simulink model "dynamicIMmodel"  (R2023b)
settings: Solver=VariableStepAuto  StartTime=0.0  StopTime=100  RelTol=1e-3
undefined symbols (not defined in the file): J, P, rr, rs, wb, Wb, We, Xlr, Xls, Xm
settings Model: Creator=Akaashdeep B  LastModifiedBy=Akaashdeep B

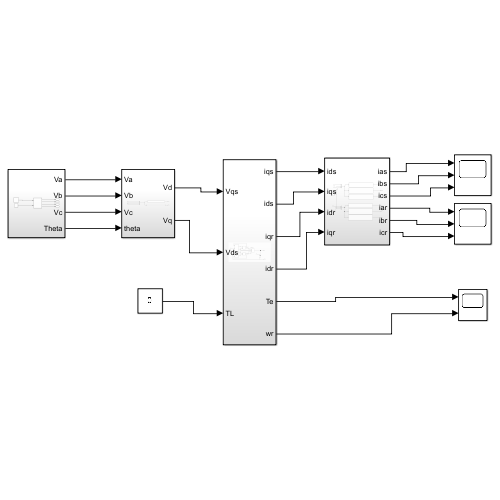
[thumbnail: Simulink's stored preview of the top-level diagram]
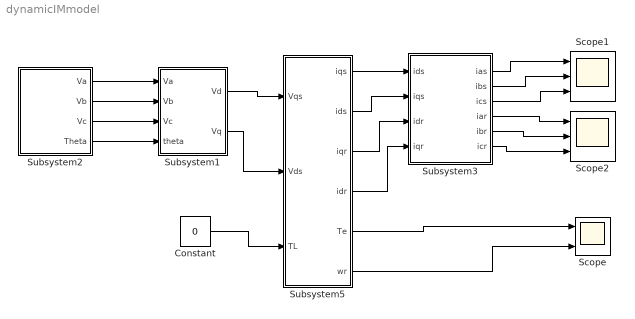
== system dynamicIMmodel ==
  Constant : Constant  Value=0
  Scope : Scope  NumInputPorts=2
  Scope1 : Scope  NumInputPorts=3
  Scope2 : Scope  NumInputPorts=3
  Subsystem1 : Subsystem
  Subsystem2 : Subsystem
  Subsystem3 : Subsystem
  Subsystem5 : Subsystem
  wires:
  Subsystem2/1(Va) -> Subsystem1/1(Va)
  Subsystem2/2(Vb) -> Subsystem1/2(Vb)
  Subsystem2/4(Theta) -> Subsystem1/4(theta)
  Subsystem1/1(Vd) -> Subsystem5/1(Vqs)
  Subsystem1/2(Vq) -> Subsystem5/2(Vds)
  Constant/1 -> Subsystem5/3(TL)
  Subsystem5/6(wr) -> Scope/2
  Subsystem5/5(Te) -> Scope/1
  Subsystem5/1(iqs) -> Subsystem3/1(ids)
  Subsystem5/2(ids) -> Subsystem3/2(iqs)
  Subsystem5/3(iqr) -> Subsystem3/3(idr)
  Subsystem5/4(idr) -> Subsystem3/4(iqr)
  Subsystem3/1(ias) -> Scope1/1
  Subsystem3/2(ibs) -> Scope1/2
  Subsystem3/3(ics) -> Scope1/3
  Subsystem3/4(iar) -> Scope2/1
  Subsystem3/5(ibr) -> Scope2/2
  Subsystem3/6(icr) -> Scope2/3
  Subsystem2/3(Vc) -> Subsystem1/3(Vc)

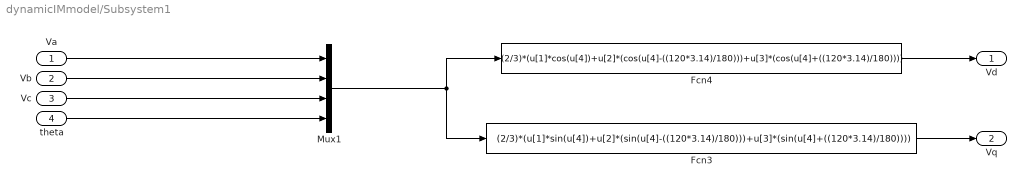
== system dynamicIMmodel/Subsystem1 ==
  Va : Inport
  Vb : Inport  Port=2
  Vc : Inport  Port=3
  theta : Inport  Port=4
  Fcn3 : Fcn  Expr=(2/3)*(u[1]*sin(u[4])+u[2]*(sin(u[4]-((120*3.14)/180)))+u[3]*(sin(u[4]+((120*3.14)/180))))
  Fcn4 : Fcn  Expr=(2/3)*(u[1]*cos(u[4])+u[2]*(cos(u[4]-((120*3.14)/180)))+u[3]*(cos(u[4]+((120*3.14)/180))))
  Mux1 : Mux
  Vd : Outport
  Vq : Outport  Port=2
  wires:
  Va/1 -> Mux1/1
  Vb/1 -> Mux1/2
  Mux1/1 -> Fcn3/1, Fcn4/1
  theta/1 -> Mux1/4
  Fcn4/1 -> Vd/1
  Vc/1 -> Mux1/3
  Fcn3/1 -> Vq/1

== system dynamicIMmodel/Subsystem2 ==
  Constant1 : Constant  Value=368.1
  Constant2 : Constant  Value=200
  Subsystem : Subsystem
  Va : Outport
  Vb : Outport  Port=2
  Vc : Outport  Port=3
  Theta : Outport  Port=4
  wires:
  Constant1/1 -> Subsystem/2(In2)
  Constant2/1 -> Subsystem/1(In1)
  Subsystem/2(Vb) -> Vb/1
  Subsystem/3(Vc) -> Vc/1
  Subsystem/4(Theta) -> Theta/1
  Subsystem/1(Va) -> Va/1

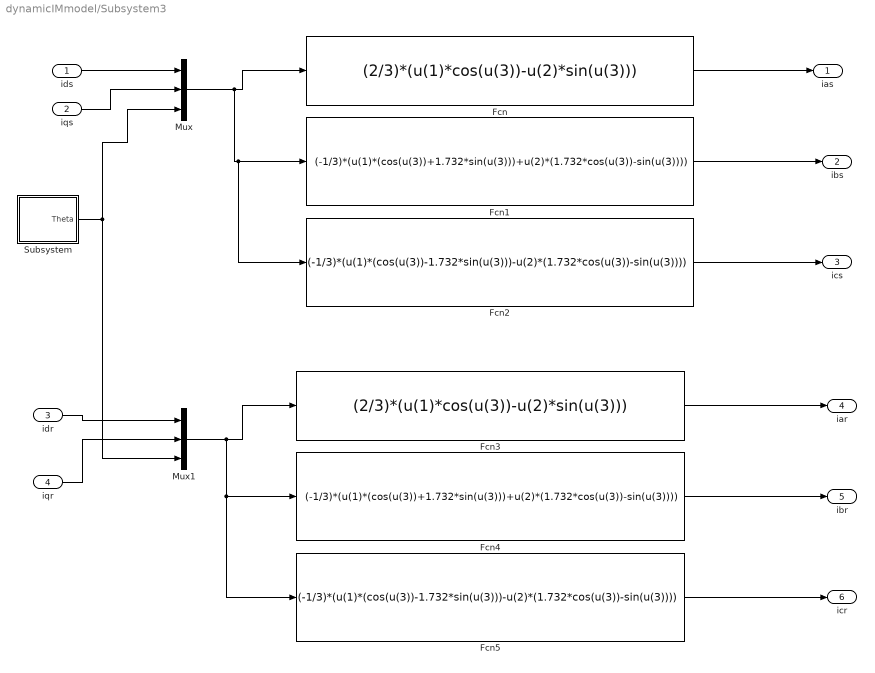
== system dynamicIMmodel/Subsystem3 ==
  ids : Inport
  iqs : Inport  Port=2
  idr : Inport  Port=3
  iqr : Inport  Port=4
  Fcn : Fcn  Expr=(2/3)*(u(1)*cos(u(3))-u(2)*sin(u(3)))
  Fcn1 : Fcn  Expr=(-1/3)*(u(1)*(cos(u(3))+1.732*sin(u(3)))+u(2)*(1.732*cos(u(3))-sin(u(3))))
  Fcn2 : Fcn  Expr=(-1/3)*(u(1)*(cos(u(3))-1.732*sin(u(3)))-u(2)*(1.732*cos(u(3))-sin(u(3))))
  Fcn3 : Fcn  Expr=(2/3)*(u(1)*cos(u(3))-u(2)*sin(u(3)))
  Fcn4 : Fcn  Expr=(-1/3)*(u(1)*(cos(u(3))+1.732*sin(u(3)))+u(2)*(1.732*cos(u(3))-sin(u(3))))
  Fcn5 : Fcn  Expr=(-1/3)*(u(1)*(cos(u(3))-1.732*sin(u(3)))-u(2)*(1.732*cos(u(3))-sin(u(3))))
  Mux : Mux  Inputs=3
  Mux1 : Mux  Inputs=3
  Subsystem : Subsystem
  ias : Outport
  ibs : Outport  Port=2
  ics : Outport  Port=3
  iar : Outport  Port=4
  ibr : Outport  Port=5
  icr : Outport  Port=6
  wires:
  Mux1/1 -> Fcn3/1, Fcn4/1, Fcn5/1
  ids/1 -> Mux/1
  Fcn5/1 -> icr/1
  idr/1 -> Mux1/1
  Fcn4/1 -> ibr/1
  Subsystem/1(Theta) -> Mux1/3, Mux/3
  Mux/1 -> Fcn2/1, Fcn1/1, Fcn/1
  Fcn2/1 -> ics/1
  iqs/1 -> Mux/2
  iqr/1 -> Mux1/2
  Fcn1/1 -> ibs/1
  Fcn/1 -> ias/1
  Fcn3/1 -> iar/1

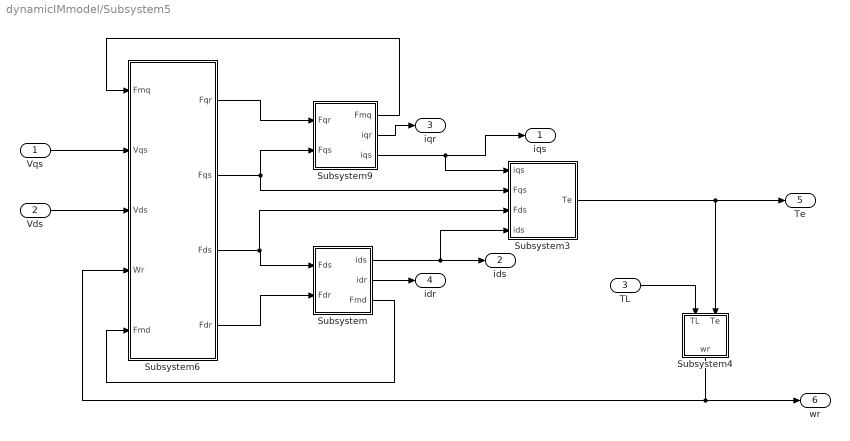
== system dynamicIMmodel/Subsystem5 ==
  Vqs : Inport
  Vds : Inport  Port=2
  TL : Inport  Port=3
  Subsystem : Subsystem
  Subsystem3 : Subsystem
  Subsystem4 : Subsystem
  Subsystem6 : Subsystem
  Subsystem9 : Subsystem
  iqs : Outport
  ids : Outport  Port=2
  iqr : Outport  Port=3
  idr : Outport  Port=4
  Te : Outport  Port=5
  wr : Outport  Port=6
  wires:
  Subsystem4/1(wr) -> wr/1, Subsystem6/4(Wr)
  Subsystem6/2(Fqs) -> Subsystem3/2(Fqs), Subsystem9/2(Fqs)
  Subsystem9/1(Fmq) -> Subsystem6/1(Fmq)
  Subsystem/2(idr) -> idr/1
  Subsystem9/3(iqs) -> iqs/1, Subsystem3/1(iqs)
  Vds/1 -> Subsystem6/3(Vds)
  Subsystem6/4(Fdr) -> Subsystem/2(Fdr)
  Vqs/1 -> Subsystem6/2(Vqs)
  Subsystem6/3(Fds) -> Subsystem3/3(Fds), Subsystem/1(Fds)
  Subsystem3/1(Te) -> Te/1, Subsystem4/2(Te)
  Subsystem9/2(iqr) -> iqr/1
  TL/1 -> Subsystem4/1(TL)
  Subsystem/1(ids) -> ids/1, Subsystem3/4(ids)
  Subsystem/3(Fmd) -> Subsystem6/5(Fmd)
  Subsystem6/1(Fqr) -> Subsystem9/1(Fqr)

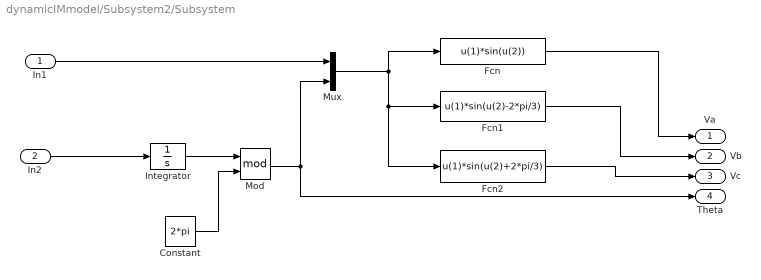
== system dynamicIMmodel/Subsystem2/Subsystem ==
  In1 : Inport
  In2 : Inport  Port=2
  Constant : Constant  Value=2*pi
  Fcn : Fcn  Expr=u(1)*sin(u(2))
  Fcn1 : Fcn  Expr=u(1)*sin(u(2)-2*pi/3)
  Fcn2 : Fcn  Expr=u(1)*sin(u(2)+2*pi/3)
  Integrator : Integrator
  Mod : Math  Operator=mod
  Mux : Mux  Inputs=2
  Va : Outport
  Vb : Outport  Port=2
  Vc : Outport  Port=3
  Theta : Outport  Port=4
  wires:
  Mod/1 -> Theta/1, Mux/2
  Constant/1 -> Mod/2
  Mux/1 -> Fcn2/1, Fcn1/1, Fcn/1
  Fcn1/1 -> Vb/1
  Integrator/1 -> Mod/1
  Fcn/1 -> Va/1
  In1/1 -> Mux/1
  Fcn2/1 -> Vc/1
  In2/1 -> Integrator/1

== system dynamicIMmodel/Subsystem3/Subsystem ==
  Constant1 : Constant  Value=2*pi
  Constant2 : Constant  Value=368.1
  Integrator : Integrator
  Mod : Math  Operator=mod
  Theta : Outport
  wires:
  Constant2/1 -> Integrator/1
  Constant1/1 -> Mod/2
  Integrator/1 -> Mod/1
  Mod/1 -> Theta/1

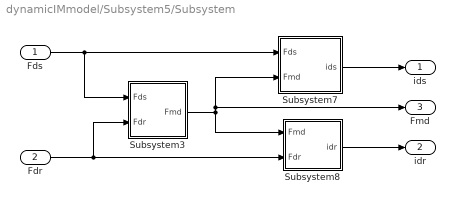
== system dynamicIMmodel/Subsystem5/Subsystem ==
  Fds : Inport
  Fdr : Inport  Port=2
  Subsystem3 : Subsystem
  Subsystem7 : Subsystem
  Subsystem8 : Subsystem
  ids : Outport
  idr : Outport  Port=2
  Fmd : Outport  Port=3
  wires:
  Subsystem3/1(Fmd) -> Fmd/1, Subsystem7/2(Fmd), Subsystem8/1(Fmd)
  Fds/1 -> Subsystem3/1(Fds), Subsystem7/1(Fds)
  Subsystem8/1(idr) -> idr/1
  Fdr/1 -> Subsystem3/2(Fdr), Subsystem8/2(Fdr)
  Subsystem7/1(ids) -> ids/1

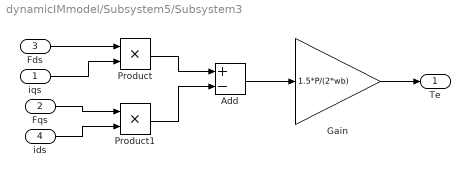
== system dynamicIMmodel/Subsystem5/Subsystem3 ==
  iqs : Inport
  Fqs : Inport  Port=2
  Fds : Inport  Port=3
  ids : Inport  Port=4
  Add : Sum  Inputs=+-
  Gain : Gain  Gain=1.5*P/(2*wb)
  Product : Product
  Product1 : Product
  Te : Outport
  wires:
  Product/1 -> Add/1
  Fqs/1 -> Product1/1
  Add/1 -> Gain/1
  Fds/1 -> Product/1
  iqs/1 -> Product/2
  ids/1 -> Product1/2
  Gain/1 -> Te/1
  Product1/1 -> Add/2

== system dynamicIMmodel/Subsystem5/Subsystem4 ==
  TL : Inport
  Te : Inport  Port=2
  Gain1 : Gain  Gain=P/(2*J)
  Integrator : Integrator
  Subtract : Sum  Inputs=+-
  wr : Outport
  wires:
  TL/1 -> Subtract/2
  Integrator/1 -> wr/1
  Subtract/1 -> Gain1/1
  Te/1 -> Subtract/1
  Gain1/1 -> Integrator/1

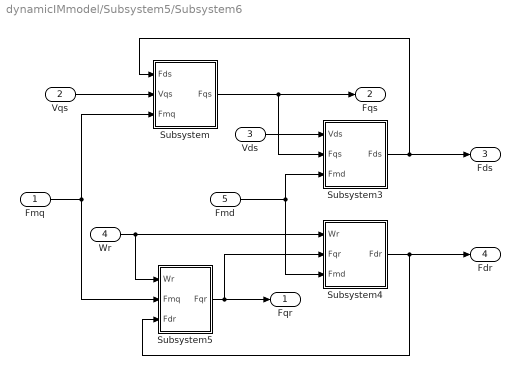
== system dynamicIMmodel/Subsystem5/Subsystem6 ==
  Fmq : Inport
  Vqs : Inport  Port=2
  Vds : Inport  Port=3
  Wr : Inport  Port=4
  Fmd : Inport  Port=5
  Subsystem : Subsystem
  Subsystem3 : Subsystem
  Subsystem4 : Subsystem
  Subsystem5 : Subsystem
  Fqr : Outport
  Fqs : Outport  Port=2
  Fds : Outport  Port=3
  Fdr : Outport  Port=4
  wires:
  Wr/1 -> Subsystem4/1(Wr), Subsystem5/1(Wr)
  Subsystem/1(Fqs) -> Fqs/1, Subsystem3/2(Fqs)
  Fmd/1 -> Subsystem4/3(Fmd), Subsystem3/3(Fmd)
  Subsystem3/1(Fds) -> Fds/1, Subsystem/1(Fds)
  Subsystem5/1(Fqr) -> Fqr/1, Subsystem4/2(Fqr)
  Vqs/1 -> Subsystem/2(Vqs)
  Fmq/1 -> Subsystem5/2(Fmq), Subsystem/3(Fmq)
  Vds/1 -> Subsystem3/1(Vds)
  Subsystem4/1(Fdr) -> Fdr/1, Subsystem5/3(Fdr)

== system dynamicIMmodel/Subsystem5/Subsystem9 ==
  Fqr : Inport
  Fqs : Inport  Port=2
  Subsystem : Subsystem
  Subsystem4 : Subsystem
  Subsystem5 : Subsystem
  Fmq : Outport
  iqr : Outport  Port=2
  iqs : Outport  Port=3
  wires:
  Subsystem4/1(iqs) -> iqs/1
  Fqs/1 -> Subsystem/1(Fqs), Subsystem4/1(Fqs)
  Subsystem5/1(iqr) -> iqr/1
  Subsystem/1(Fmq) -> Fmq/1, Subsystem4/2(Fmq), Subsystem5/1(Fmq)
  Fqr/1 -> Subsystem/2(Fqr), Subsystem5/2(Fqr)

== system dynamicIMmodel/Subsystem5/Subsystem/Subsystem3 ==
  Fds : Inport
  Fdr : Inport  Port=2
  Gain : Gain  Gain=1/Xls
  Gain1 : Gain  Gain=1/Xlr
  Gain2 : Gain  Gain=1/((1/Xm)+(1/Xls)+(1/Xlr))
  Sum : Sum
  Fmd : Outport
  wires:
  Gain2/1 -> Fmd/1
  Gain1/1 -> Sum/2
  Fdr/1 -> Gain1/1
  Gain/1 -> Sum/1
  Fds/1 -> Gain/1
  Sum/1 -> Gain2/1

== system dynamicIMmodel/Subsystem5/Subsystem/Subsystem7 ==
  Fds : Inport
  Fmd : Inport  Port=2
  Add : Sum  Inputs=+-
  Gain : Gain  Gain=1/Xls
  ids : Outport
  wires:
  Gain/1 -> ids/1
  Fmd/1 -> Add/2
  Add/1 -> Gain/1
  Fds/1 -> Add/1

== system dynamicIMmodel/Subsystem5/Subsystem/Subsystem8 ==
  Fmd : Inport
  Fdr : Inport  Port=2
  Add1 : Sum  Inputs=-+
  Gain1 : Gain  Gain=1/Xlr
  idr : Outport
  wires:
  Fmd/1 -> Add1/1
  Add1/1 -> Gain1/1
  Fdr/1 -> Add1/2
  Gain1/1 -> idr/1

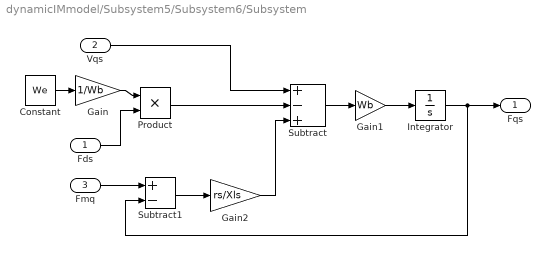
== system dynamicIMmodel/Subsystem5/Subsystem6/Subsystem ==
  Fds : Inport
  Vqs : Inport  Port=2
  Fmq : Inport  Port=3
  Constant : Constant  Value=We
  Gain : Gain  Gain=1/Wb
  Gain1 : Gain  Gain=Wb
  Gain2 : Gain  Gain=rs/Xls
  Integrator : Integrator
  Product : Product
  Subtract : Sum  Inputs=+-+
  Subtract1 : Sum  Inputs=+-
  Fqs : Outport
  wires:
  Gain/1 -> Product/1
  Product/1 -> Subtract/2
  Integrator/1 -> Fqs/1, Subtract1/2
  Fds/1 -> Product/2
  Fmq/1 -> Subtract1/1
  Vqs/1 -> Subtract/1
  Subtract/1 -> Gain1/1
  Constant/1 -> Gain/1
  Gain2/1 -> Subtract/3
  Subtract1/1 -> Gain2/1
  Gain1/1 -> Integrator/1

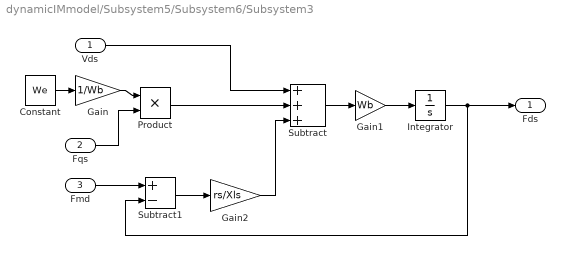
== system dynamicIMmodel/Subsystem5/Subsystem6/Subsystem3 ==
  Vds : Inport
  Fqs : Inport  Port=2
  Fmd : Inport  Port=3
  Constant : Constant  Value=We
  Gain : Gain  Gain=1/Wb
  Gain1 : Gain  Gain=Wb
  Gain2 : Gain  Gain=rs/Xls
  Integrator : Integrator
  Product : Product
  Subtract : Sum  Inputs=+++
  Subtract1 : Sum  Inputs=+-
  Fds : Outport
  wires:
  Subtract/1 -> Gain1/1
  Integrator/1 -> Fds/1, Subtract1/2
  Gain/1 -> Product/1
  Product/1 -> Subtract/2
  Gain1/1 -> Integrator/1
  Vds/1 -> Subtract/1
  Subtract1/1 -> Gain2/1
  Gain2/1 -> Subtract/3
  Fqs/1 -> Product/2
  Constant/1 -> Gain/1
  Fmd/1 -> Subtract1/1

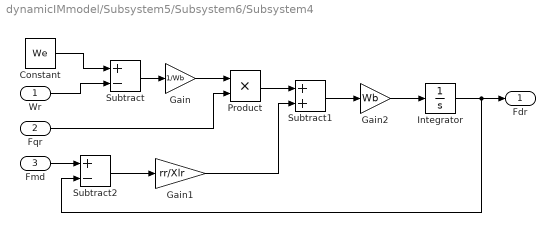
== system dynamicIMmodel/Subsystem5/Subsystem6/Subsystem4 ==
  Wr : Inport
  Fqr : Inport  Port=2
  Fmd : Inport  Port=3
  Constant : Constant  Value=We
  Gain : Gain  Gain=1/Wb
  Gain1 : Gain  Gain=rr/Xlr
  Gain2 : Gain  Gain=Wb
  Integrator : Integrator
  Product : Product
  Subtract : Sum  Inputs=+-
  Subtract1 : Sum
  Subtract2 : Sum  Inputs=+-
  Fdr : Outport
  wires:
  Gain1/1 -> Subtract1/2
  Integrator/1 -> Subtract2/2, Fdr/1
  Gain/1 -> Product/1
  Fmd/1 -> Subtract2/1
  Subtract/1 -> Gain/1
  Subtract1/1 -> Gain2/1
  Gain2/1 -> Integrator/1
  Constant/1 -> Subtract/1
  Product/1 -> Subtract1/1
  Subtract2/1 -> Gain1/1
  Fqr/1 -> Product/2
  Wr/1 -> Subtract/2

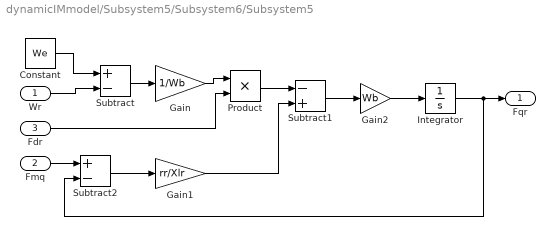
== system dynamicIMmodel/Subsystem5/Subsystem6/Subsystem5 ==
  Wr : Inport
  Fmq : Inport  Port=2
  Fdr : Inport  Port=3
  Constant : Constant  Value=We
  Gain : Gain  Gain=1/Wb
  Gain1 : Gain  Gain=rr/Xlr
  Gain2 : Gain  Gain=Wb
  Integrator : Integrator
  Product : Product
  Subtract : Sum  Inputs=+-
  Subtract1 : Sum  Inputs=-+
  Subtract2 : Sum  Inputs=+-
  Fqr : Outport
  wires:
  Subtract2/1 -> Gain1/1
  Subtract1/1 -> Gain2/1
  Subtract/1 -> Gain/1
  Fmq/1 -> Subtract2/1
  Gain1/1 -> Subtract1/2
  Gain/1 -> Product/1
  Integrator/1 -> Subtract2/2, Fqr/1
  Product/1 -> Subtract1/1
  Constant/1 -> Subtract/1
  Wr/1 -> Subtract/2
  Fdr/1 -> Product/2
  Gain2/1 -> Integrator/1

== system dynamicIMmodel/Subsystem5/Subsystem9/Subsystem ==
  Fqs : Inport
  Fqr : Inport  Port=2
  Gain : Gain  Gain=1/Xls
  Gain1 : Gain  Gain=1/Xlr
  Gain2 : Gain  Gain=1/((1/Xm)+(1/Xls)+(1/Xlr))
  Sum : Sum
  Fmq : Outport
  wires:
  Gain1/1 -> Sum/2
  Sum/1 -> Gain2/1
  Gain2/1 -> Fmq/1
  Gain/1 -> Sum/1
  Fqr/1 -> Gain1/1
  Fqs/1 -> Gain/1

== system dynamicIMmodel/Subsystem5/Subsystem9/Subsystem4 ==
  Fqs : Inport
  Fmq : Inport  Port=2
  Add : Sum  Inputs=+-
  Gain : Gain  Gain=1/Xls
  iqs : Outport
  wires:
  Fqs/1 -> Add/1
  Add/1 -> Gain/1
  Fmq/1 -> Add/2
  Gain/1 -> iqs/1

== system dynamicIMmodel/Subsystem5/Subsystem9/Subsystem5 ==
  Fmq : Inport
  Fqr : Inport  Port=2
  Add1 : Sum  Inputs=-+
  Gain1 : Gain  Gain=1/Xlr
  iqr : Outport
  wires:
  Gain1/1 -> iqr/1
  Fqr/1 -> Add1/2
  Add1/1 -> Gain1/1
  Fmq/1 -> Add1/1
